simulink library "variableFlowProfileCalculationYZ_ul"  (R2018b)
settings: Solver=VariableStepAuto  StartTime=0.0  StopTime=10.0  RelTol=1e-3
libraries: dspmtrx3 x5, Dynamic_2D_Lookup_Table x3
settings Model: Creator=James Reed  LastModifiedBy=jcreed2

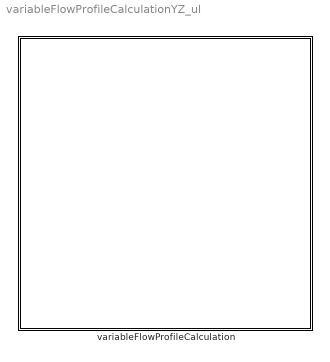
== system variableFlowProfileCalculationYZ_ul ==
  variableFlowProfileCalculation : Subsystem

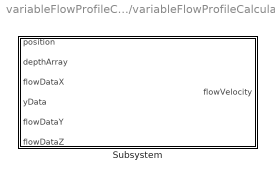
== system variableFlowProfileCalculationYZ_ul/variableFlowProfileCalculation ==
  Subsystem : Subsystem

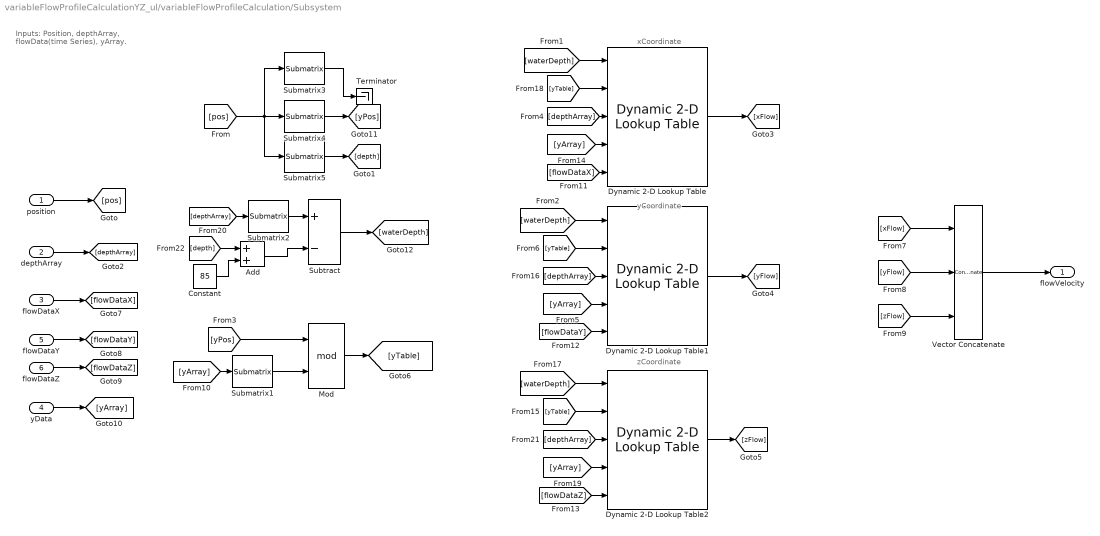
== system variableFlowProfileCalculationYZ_ul/variableFlowProfileCalculation/Subsystem ==
  note: Inputs: Position, depthArray,
      | flowData(time Series), yArray.
  note: xCoordinate
  note: zCoordinate
  note: yCoordinate
  "position " : Inport
  "depthArray " : Inport  Port=2
  "flowDataX " : Inport  Port=3
  "yData " : Inport  Port=4
  "flowDataY " : Inport  Port=5
  flowDataZ : Inport  Port=6
  Add : Sum
  Constant : Constant  Value=85
  Dynamic 2-D Lookup Table : Dynamic_2D_Lookup_Table/Dynamic 2-D Lookup Table
  Dynamic 2-D Lookup Table1 : Dynamic_2D_Lookup_Table/Dynamic 2-D Lookup Table
  Dynamic 2-D Lookup Table2 : Dynamic_2D_Lookup_Table/Dynamic 2-D Lookup Table
  Mod : Math  Operator=mod  SaturateOnIntegerOverflow=on
  Submatrix1 : dspmtrx3/Submatrix  RowSpan=One row  RowStartMode=Last  RowStartIndex=1  RowEndMode=Last  RowEndIndex=1  ColSpan=All columns  ColStartMode=Last  ColStartIndex=1  ColEndMode=Last  ColEndIndex=1
  Submatrix2 : dspmtrx3/Submatrix  RowSpan=One row  RowStartMode=Last  RowStartIndex=1  RowEndMode=Last  RowEndIndex=1  ColSpan=All columns  ColStartMode=Last  ColStartIndex=1  ColEndMode=Last  ColEndIndex=1
  Submatrix3 : dspmtrx3/Submatrix  RowSpan=One row  RowStartMode=First  RowStartIndex=1  RowEndMode=Last  RowEndIndex=1  ColSpan=All columns  ColStartMode=First  ColStartIndex=1  ColEndMode=Last  ColEndIndex=1
  Submatrix4 : dspmtrx3/Submatrix  RowSpan=One row  RowStartMode=First  RowStartIndex=1  RowEndMode=Last  RowEndIndex=1  ColSpan=All columns  ColStartMode=First  ColStartIndex=1  ColEndMode=Last  ColEndIndex=1
  Submatrix5 : dspmtrx3/Submatrix  RowSpan=One row  RowStartMode=First  RowStartIndex=1  RowEndMode=Last  RowEndIndex=1  ColSpan=All columns  ColStartMode=First  ColStartIndex=1  ColEndMode=Last  ColEndIndex=1
  Subtract : Sum  Inputs=+-
  Terminator : Terminator
  Vector Concatenate : Concatenate  NumInputs=3  Mode=Multidimensional array
  "flowVelocity " : Outport
  wires:
  Dynamic 2-D Lookup Table2/1 -> [zFlow]
  [yArray] -> Dynamic 2-D Lookup Table/4
  Dynamic 2-D Lookup Table1/1 -> [yFlow]
  [waterDepth] -> Dynamic 2-D Lookup Table1/1
  [yTable] -> Dynamic 2-D Lookup Table1/2
  [xFlow] -> Vector Concatenate/1
  Dynamic 2-D Lookup Table/1 -> [xFlow]
  Submatrix3/1 -> Terminator/1
  [flowDataY] -> Dynamic 2-D Lookup Table1/5
  Vector Concatenate/1 -> "flowVelocity "/1
  [zFlow] -> Vector Concatenate/3
  [pos] -> Submatrix3/1, Submatrix5/1, Submatrix4/1
  [waterDepth] -> Dynamic 2-D Lookup Table/1
  [depthArray] -> Dynamic 2-D Lookup Table2/3
  [waterDepth] -> Dynamic 2-D Lookup Table2/1
  [flowDataZ] -> Dynamic 2-D Lookup Table2/5
  "yData "/1 -> [yArray]
  [yArray] -> Dynamic 2-D Lookup Table2/4
  [depthArray] -> Dynamic 2-D Lookup Table1/3
  [yArray] -> Dynamic 2-D Lookup Table1/4
  [yTable] -> Dynamic 2-D Lookup Table2/2
  "flowDataX "/1 -> [flowDataX]
  "position "/1 -> [pos]
  Submatrix4/1 -> [yPos]
  [yTable] -> Dynamic 2-D Lookup Table/2
  "depthArray "/1 -> [depthArray]
  [depthArray] -> Dynamic 2-D Lookup Table/3
  Submatrix5/1 -> [depth]
  [yFlow] -> Vector Concatenate/2
  [flowDataX] -> Dynamic 2-D Lookup Table/5
  "flowDataY "/1 -> [flowDataY]
  flowDataZ/1 -> [flowDataZ]
  [yPos] -> Mod/1
  Submatrix1/1 -> Mod/2
  [yArray] -> Submatrix1/1
  Mod/1 -> [yTable]
  [depth] -> Add/1
  Subtract/1 -> [waterDepth]
  [depthArray] -> Submatrix2/1
  Submatrix2/1 -> Subtract/1
  Constant/1 -> Add/2
  Add/1 -> Subtract/2
